simulink model "ITRI_Block_PDFF_Ccode_XZ"  (R2017b)
settings: Solver=VariableStepAuto  StartTime=0.0  StopTime=Reference_time  RelTol=1e-3
values from neighbouring files (symbols this model uses):
  F_x = 1    [mainA_itri_pdff.m]
  F_z = 1    [mainA_itri_pdff.m]
  Kd_x = 0.090865    [mainA_itri_pdff.m]
  Kd_z = 0.14788    [mainA_itri_pdff.m]
  Kp_x = 65.4554    [mainA_itri_pdff.m]
  Kp_z = 66.0566    [mainA_itri_pdff.m]
  Ts = 0.001    [ID_Model_ITRI.m]
libraries: cstblocks x2, slctrlblks x1
settings Model: Creator=LAB816  LastModifiedBy=LAB_JHU

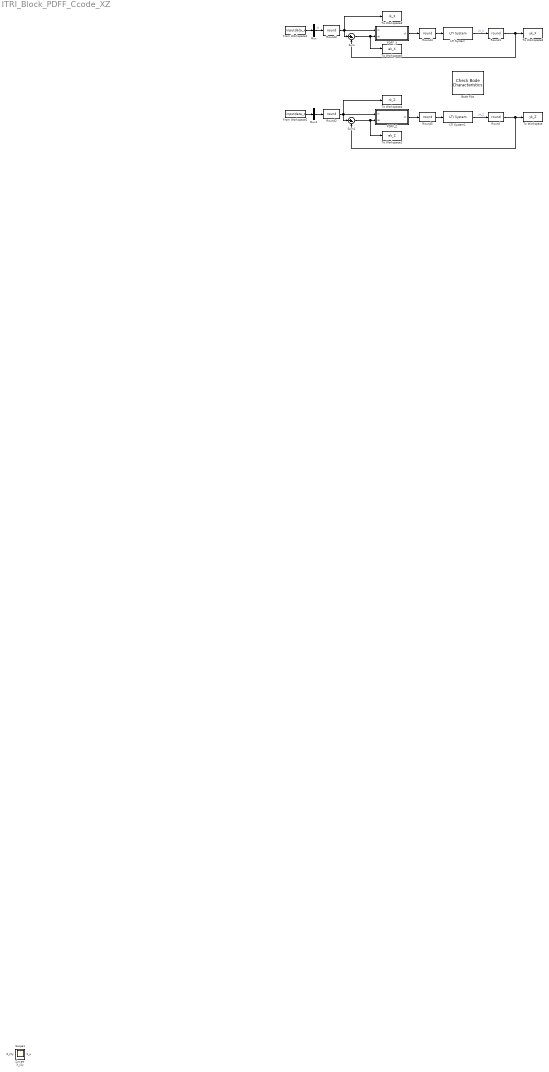
== system ITRI_Block_PDFF_Ccode_XZ ==
  Bode Plot : slctrlblks/Model Verification/Check Bode  Characteristics  InstantiateOnLoad=on  SaveOperatingPoints=off  LinearizationIOs={'/Round', 1, 'outin', 'off', ''}  LinearizeAt=SnapshotTimes  SnapshotTimes=[0]  TriggerType=rising  SampleTime=auto  RateConversionMethod=zoh  PreWarpFreq=10  UseExactDelayModel=off  UseFullBlockNameLabels=off  UseBusSignalLabels=off  enabled=on  stopWhenAssertionFail=off  export=off  ViewDlgPos=[102 200 508 390]  OpenViewOnLoad=off  LaunchViewOnOpen=on  FrequencyUnits=rad/s  MagnitudeUnits=dB  PhaseUnits=deg  TimeUnits=seconds  EnableUpperBound=off  UpperBoundFrequencies=[]  UpperBoundMagnitudes=[]  EnableLowerBound=off  LowerBoundFrequencies=[]  LowerBoundMagnitudes=[]
      settings: SourceProductName=Simulink Control Design
  From Workspace1 : FromWorkspace  VariableName=inputdata_x  SampleTime=Ts
  From Workspace2 : FromWorkspace  VariableName=inputdata_z  SampleTime=Ts
  LTI System : cstblocks/LTI System  sys=plantX_ITRI.v2p  IC=[]
  LTI System1 : cstblocks/LTI System  sys=plantZ_ITRI.v2p  IC=[]
  Mux : Mux  Inputs=1
  Mux1 : Mux  Inputs=1
  PDFF_X : Subsystem
  PDFF_Z : Subsystem
  Round{,1..5} (6 alike) : Rounding  Operator=round
  Sum : Sum  Inputs=|+-
  Sum1 : Sum  Inputs=|+-
  To Workspace : ToWorkspace  VariableName=yk_Z  SampleTime=-1
  To Workspace1 : ToWorkspace  VariableName=ek_Z  SampleTime=-1
  To Workspace2 : ToWorkspace  VariableName=yk_X  SampleTime=-1
  To Workspace3 : ToWorkspace  VariableName=rk_X  SampleTime=-1
  To Workspace4 : ToWorkspace  VariableName=rk_Z  SampleTime=-1
  To Workspace5 : ToWorkspace  VariableName=ek_X  SampleTime=-1
  Scope : Scope
  Scope1 : Scope
  X_r2y : Scope
  X_u : Scope
  Z_r2y : Scope
  Z_u : Scope
  wires:
  PDFF_X/1(uk) -> Round4/1
  Mux/1 -> Round3/1  "rk"
  LTI System/1 -> Round1/1  "yk_X"
  LTI System1/1 -> Round/1  "yk_Z"
  From Workspace1/1 -> Mux/1
  Sum1/1 -> To Workspace1/1, PDFF_Z/2(ek)
  PDFF_Z/1(uk) -> Round5/1
  Sum/1 -> To Workspace5/1, PDFF_X/2(ek)
  Mux1/1 -> Round2/1
  From Workspace2/1 -> Mux1/1
  Round/1 -> To Workspace/1, Sum1/2
  Round1/1 -> To Workspace2/1, Sum/2
  Round2/1 -> Sum1/1, To Workspace4/1, PDFF_Z/1(rk)
  Round3/1 -> Sum/1, PDFF_X/1(rk), To Workspace3/1
  Round4/1 -> LTI System/1
  Round5/1 -> LTI System1/1

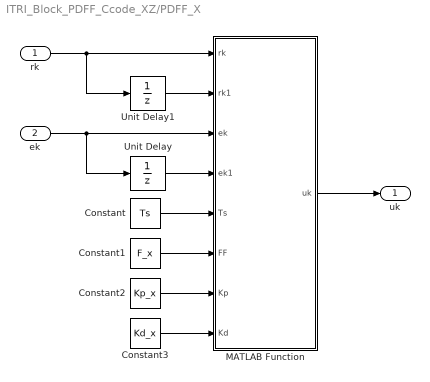
== system ITRI_Block_PDFF_Ccode_XZ/PDFF_X ==
  rk : Inport
  ek : Inport  Port=2
  Constant : Constant  Value=Ts
  Constant1 : Constant  Value=F_x
  Constant2 : Constant  Value=Kp_x
  Constant3 : Constant  Value=Kd_x
  MATLAB Function : MATLAB Function  TreatAsAtomicUnit=on
  Unit Delay : UnitDelay  SampleTime=-1
  Unit Delay1 : UnitDelay  SampleTime=-1
  uk : Outport
  wires:
  Constant3/1 -> MATLAB Function/8(Kd)
  Constant2/1 -> MATLAB Function/7(Kp)
  Constant1/1 -> MATLAB Function/6(FF)
  ek/1 -> MATLAB Function/3(ek), Unit Delay/1
  rk/1 -> MATLAB Function/1(rk), Unit Delay1/1
  MATLAB Function/1(uk) -> uk/1
  Unit Delay/1 -> MATLAB Function/4(ek1)
  Unit Delay1/1 -> MATLAB Function/2(rk1)
  Constant/1 -> MATLAB Function/5(Ts)

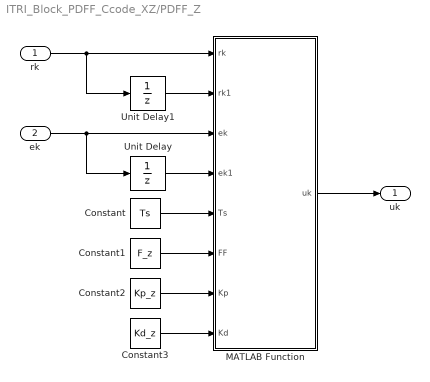
== system ITRI_Block_PDFF_Ccode_XZ/PDFF_Z ==
  rk : Inport
  ek : Inport  Port=2
  Constant : Constant  Value=Ts
  Constant1 : Constant  Value=F_z
  Constant2 : Constant  Value=Kp_z
  Constant3 : Constant  Value=Kd_z
  MATLAB Function : MATLAB Function  TreatAsAtomicUnit=on
  Unit Delay : UnitDelay  SampleTime=-1
  Unit Delay1 : UnitDelay  SampleTime=-1
  uk : Outport
  wires:
  Constant/1 -> MATLAB Function/5(Ts)
  Unit Delay1/1 -> MATLAB Function/2(rk1)
  Unit Delay/1 -> MATLAB Function/4(ek1)
  MATLAB Function/1(uk) -> uk/1
  rk/1 -> Unit Delay1/1, MATLAB Function/1(rk)
  ek/1 -> Unit Delay/1, MATLAB Function/3(ek)
  Constant1/1 -> MATLAB Function/6(FF)
  Constant2/1 -> MATLAB Function/7(Kp)
  Constant3/1 -> MATLAB Function/8(Kd)

== matlab function ITRI_Block_PDFF_Ccode_XZ/PDFF_X/MATLAB Function ==
  data: rk input; uk output; rk1 input; ek input; ek1 input; Ts input; FF input; Kp input; Kd input
function uk = PDFF_x(rk,rk1,ek,ek1,Ts,FF,Kp,Kd)    
    uk = FF*(rk-rk1)/Ts + Kp*ek + Kd*(ek-ek1)/Ts;
end

== matlab function ITRI_Block_PDFF_Ccode_XZ/PDFF_Z/MATLAB Function ==
  data: rk input; uk output; rk1 input; ek input; ek1 input; Ts input; FF input; Kp input; Kd input
function uk = PDFF_z(rk,rk1,ek,ek1,Ts,FF,Kp,Kd)    
    uk = FF*(rk-rk1)/Ts + Kp*ek + Kd*(ek-ek1)/Ts;
end
